simulink model "MCLV2_dsPIC33EP256MC506_externalOpAmp_DataLog"  (Simulink 9.2)
settings: Solver=FixedStepDiscrete  StartTime=0.0  StopTime=inf  FixedStep=Ts  RelTol=1e-3  EnableMultiTasking=on
PreLoadFcn:
  | InitTPV0;
undefined symbols (not defined in the file or in its folder): A4, A8, C5, C6, D5, F1, Lignes, NumBits1, NumBits2, P20, P24, P53, P54, P97, Pin, PWMmax, Slope1, Slope2, Timer, Tm, TPWM, TsQEI
undefined symbols (not defined in the file): Ts
libraries: simulink x16, MCHP_Blockset x14, simulink_need_slupdate x4, sl_helperblocks x1
(part 2 of 2)

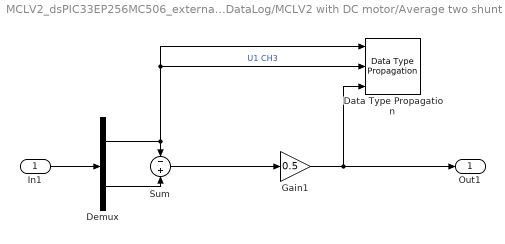
== system MCLV2_dsPIC33EP256MC506_externalOpAmp_DataLog/MCLV2 with DC motor/Average two shunt resistors ==
  In1 : Inport
  Data Type Propagation : simulink/Signal Attributes/Data Type Propagation  PropDataType=fixdt(1, 16)  IfRefDouble=double  IfRefSingle=single  IsSigned=IsSigned1 or IsSigned2  NumBitsBase=max([NumBits1 NumBits2])  NumBitsMult=1  NumBitsAdd=0  NumBitsAllowFinal=1:128  PropScaling=2^-10  ValuesUsedBestPrec=[5 -7]  SlopeBase=min([Slope1 Slope2])  SlopeMult=1  SlopeAdd=0  BiasBase=Bias1  BiasMult=1  BiasAdd=0
      settings: SourceProductName=Simulink  SourceProductBaseCode=SL
  Demux : Demux  Outputs=2
  Gain1 : Gain  Gain=0.5  ParamMin=[0.5]  ParamMax=[0.5]  OutDataTypeStr=Inherit: Inherit via back propagation  SaturateOnIntegerOverflow=on
  Sum : Sum  Inputs=-+  OutDataTypeStr=Inherit: Same as accumulator  SaturateOnIntegerOverflow=on
  Out1 : Outport
  wires:
  Demux/2 -> Sum/2
  Sum/1 -> Gain1/1
  Demux/1 -> Data Type Propagation/2, Data Type Propagation/1, Sum/1  "U1 CH3"
  In1/1 -> Demux/1
  Gain1/1 -> Data Type Propagation/3, Out1/1

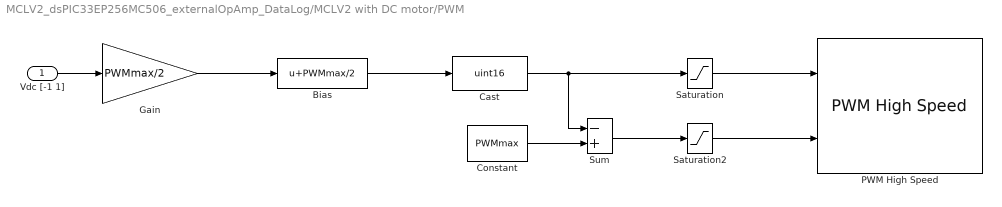
== system MCLV2_dsPIC33EP256MC506_externalOpAmp_DataLog/MCLV2 with DC motor/PWM ==
  Vdc [-1 1] : Inport
  Bias : Bias  Bias=PWMmax/2
  Cast : DataTypeConversion  OutDataTypeStr=uint16
  Constant : Constant  Value=PWMmax  OutDataTypeStr=uint16
  Gain : Gain  Gain=PWMmax/2  OutDataTypeStr=fixdt(1,32,1)
  PWM High Speed : MCHP_Blockset/PWM IO/PWM High Speed  pop1=[1]  chk1="[1  1  1  0  0]"  chkHL1="[1  1  0  1  1  1  1 ; 1  1  0  1  1  1  1]"  maxP1={ 'TPWM','0.001','0.001','0.001','0.001','0.001','0.001';'0.001','0.001','1e-06','0.001','0.001','0.001','0.001'}  InitP2={ 'TPWM','0.001','0.001','0.001','0.001','0.001','0.001';'0.001','0.001','0.001','0.001','0.001','0.001','0.001'}  chkP2="[0  1  0  1  1  1  1 ; 1  0  0  1  1  1  1]"  InitDC={ '50','50','50','50','50','50','50';'0.001','0.001','0.001','50','50','50','50'}  chkDC="[1  1  1  1  1  1  1 ; 0  0  0  1  1  1  1]"  InitPh={ '0','0','0','0.001','0.001','0.001','0.001';'0','0','0','0.001','0.001','0.001','0.001'}  chkPh="[0  0  0  1  1  1  1 ; 0  0  0  1  1  1  1]"  edSEvTrigx={ '0','-1','-1','-1','-1','-1','-1'}  chkSEvTrigx="[0  1  1  1  1  1  1]"  popFlt="[2  2  1  1  1  1  1]"  popFltPin="[20  20  20   4   4   4   4]"  popFltPinRp="[1  1  1  1  1  1  1]"  popFltActivH="[2  2  1  1  1  1  1]"  popFltForceH="[2  2  2  2  2  2  2]"  popFltForceL="[1  1  1  1  1  1  1]"  chkFltBlkOut="[0  0  0  0  0  0  0]"  popIndepFaultMode="[1  1  1  1  1  1  1]"  popCurEnabled="[1  1  1  1  1  1  1]"  popCurPin="[4  31   4   4   4   4   4]"  popCurActiveH="[1  1  1  1  1  1  1]"  popCurForceH="[2  1  2  1  1  1  1]"  popCurForceL="[2  1  2  1  1  1  1]"  ChkCurBlkOut="[1  0  0  0  0  0  0]"  ChkCurBlkOutTime="[1  0  1  0  0  0  0]"  popBLANKSEL="[1  1  1  1  1  1  1]"  popBPHHBPHL="[1  1  1  1  1  1  1]"  popBPLHBPLL="[1  1  1  1  1  1  1]"  popFLTLEBEN_CLLEBEN="[1  1  1  1  1  1  1]"  popPHR_PHF="[2  1  1  1  1  1  1]"  popPLR_PLF="[3  1  1  1  1  1  1]"  edLEB={ '100e-9','50e-9','150e-9','50e-9','50e-9','50e-9','50e-9'}  popDT="[1  1  1  3  3  3  3]"  edDTRx={ '0.02','1e-05','0.001','1e-05','1e-05','1e-05','1e-05'}  edAltDTRx={ 'Tm','Tm','Tm','1e-05','1e-05','1e-05','1e-05'}  S_INPUT="[5  5  5]"  S_INPUT_Size="[1  1  1]"  S_OUTPUT=[]  S_OUTPUT_Size=[]  S_DWORK_Type=[]  S_DWORK_Size=[]  ADC_VARTRIG={PWM Primary Special Event Trigger;6}  SampleTime=-1  ORDERING=None  MCHP_PORT={PWM1 Fault}{FLT32}4:0:B4;{PWM2 Fault}{FLT32}4:0:B4;{PWM1H}{PWM1H}4:4:B14;{PWM1L}{PWM1L}4:4:B15;{PWM2H}{PWM2H}4:4:B12;{PWM2L}{PWM2L}4:4:B13;  MCHP_MASTERLINK=MCLV2_dsPIC33EP256MC506_externalOpAmp_DataLog/Microchip Master  MCHP_VERSION=v3.39
      settings: SourceProductName=MPLAB® Device Blocks for Simulink®
  Saturation : Saturate  UpperLimit=PWMmax  LowerLimit=round( (Tm/TPWM) *PWMmax )
  Saturation2 : Saturate  UpperLimit=PWMmax  LowerLimit=round( (Tm/TPWM) *PWMmax )
  Sum : Sum  Inputs=-+  OutDataTypeStr=Inherit: Same as first input
  wires:
  Gain/1 -> Bias/1
  Cast/1 -> Sum/1, Saturation/1
  Saturation/1 -> PWM High Speed/1
  Sum/1 -> Saturation2/1
  Bias/1 -> Cast/1
  Saturation2/1 -> PWM High Speed/2
  Vdc [-1 1]/1 -> Gain/1
  Constant/1 -> Sum/2

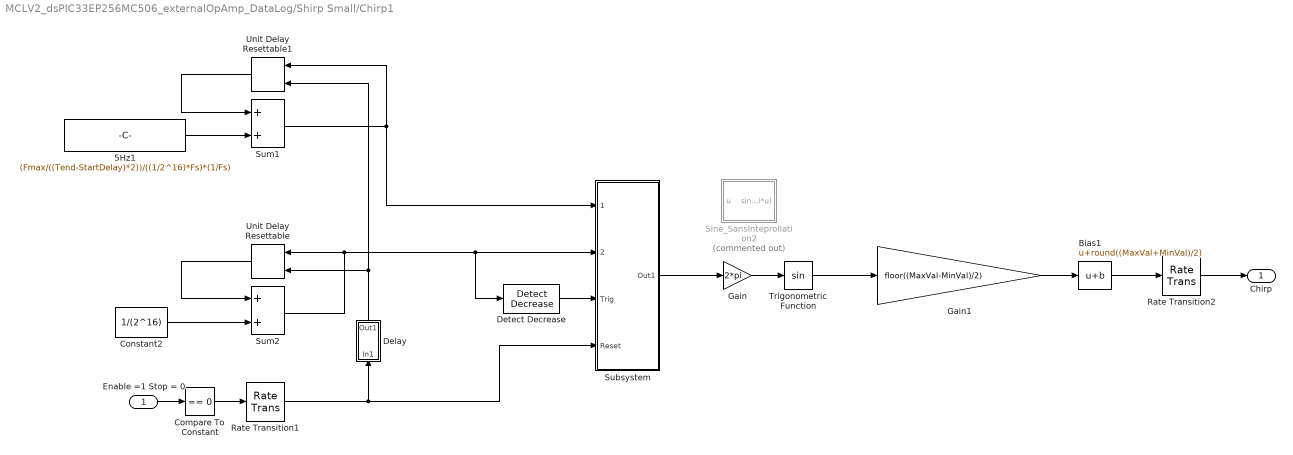
== system MCLV2_dsPIC33EP256MC506_externalOpAmp_DataLog/Shirp Small/Chirp1 ==
  Enable =1 Stop = 0 : Inport
  5Hz1 : Constant  Value=(Fmax/((Tend-StartDelay)*2))/((1/2^16)*Fs)*(1/Fs)  OutMin=(Fmax/((Tend-StartDelay)*2))/((1/2^16)*Fs)  OutMax=(Fmax/((Tend-StartDelay)*2))/((1/2^16)*Fs)  OutDataTypeStr=fixdt(0,32)  SampleTime=1/Fs
  Bias1 : Bias  Bias=round((MaxVal+MinVal)/2)
  Compare To Constant : simulink/Logic and Bit Operations/Compare To Constant  relop===  const=0  OutDataTypeStr=boolean
  Constant2 : Constant  Value=1/(2^16)  OutDataTypeStr=Inherit: Inherit via back propagation  SampleTime=1/Fs
  Delay : Subsystem
  Detect Decrease : simulink/Logic and Bit Operations/Detect Decrease  vinit=0.0  OutDataTypeStr=uint8
  Gain : Gain  Gain=2*pi  OutDataTypeStr=fixdt(0,16,13)
  Gain1 : Gain  Gain=floor((MaxVal-MinVal)/2)  OutMin=[MinVal]  OutMax=[MaxVal]  OutDataTypeStr=fixdt(MinVal<0,16)
  Rate Transition1 : RateTransition  Integrity=off  Deterministic=off
  Rate Transition2 : RateTransition  Integrity=off  Deterministic=off
  Sine_SansInteprollation2 : Subsystem  Commented=on  TreatAsAtomicUnit=on  mask(Sine and Cosine){Formula=sin(2*pi*u), NumDataPoints=(2^10)+1, OutputWordLength=16}
      mask prompts: Formula "Output formula"; NumDataPoints "Number of data points for lookup table:"; OutputWordLength "Output word length:"
      mask help:
      | Implement sine and cosine functions in fixed point using a lookup table approach that exploits quarter wave symmetry. The output fraction length equals the output word length minus 2.
      |
      | The most efficient implementation is obtained when the number of data points is (2^n)+1 where n is an integer.
      mask init:
      | if (~isnumeric(OutputWordLength)) || ( length(OutputWordLength) > 1 ) || ( OutputWordLength < 2 ) || ( floor(OutputWordLength) ~= OutputWordLength )
      |     error(DAStudio.message('Simulink:blocks:SineLookupWordLengthTooSmall'));
      | end
      | if (~isnumeric(NumDataPoints)) || ( length(NumDataPoints) > 1 ) || ( NumDataPoints < 2 ) || ( floor(NumDataPoints) ~= NumDataPoints )
      |     error(DAStudio.message('Simulink:blocks:SineLookupNumDataPtsTooSmall'));
      | end
      | if ( 2^(OutputWordLength-2) + 1 ) < NumDataPoints
      |     smallEnoughNumDataPoints = ( 2^(OutputWordLength-2) + 1 );
      |     bigEnoughOutputWordLength = ceil(log2(NumDataPoints-1))+2;
      |     error(DAStudio.message('Simulink:blocks:SineLookupEitherTooSmall',...
      |         NumDataPoints, ...
      |         smallEnoughNumDataPoints, ...
      |         OutputWordLength, ...
      |         bigEnoughOutputWordLength));
      | end
      | slsincos(Formula);
      mask TypeOptions Formula: sin(2*pi*u) | cos(2*pi*u) | exp(j*2*pi*u) | sin(2*pi*u) and cos(2*pi*u)
  Subsystem : Subsystem
  Sum1 : Sum  OutDataTypeStr=Inherit: Inherit via back propagation
  Sum2 : Sum  OutDataTypeStr=fixdt(0,16,16)
  Trigonometric Function : Trigonometry  ApproximationMethod=CORDIC
  Unit Delay Resettable : simulink_need_slupdate/Unit Delay Resettable  vinit=0.0  tsamp=inv(Fs)
      settings: SourceProductName=Simulink  SourceProductBaseCode=SL
  Unit Delay Resettable1 : simulink_need_slupdate/Unit Delay Resettable  vinit=0.0  tsamp=inv(Fs)
      settings: SourceProductName=Simulink  SourceProductBaseCode=SL
  Chirp : Outport
  wires:
  Gain/1 -> Trigonometric Function/1
  Trigonometric Function/1 -> Gain1/1
  Rate Transition1/1 -> Delay/1(In1), Subsystem/4(Reset)
  Rate Transition2/1 -> Chirp/1
  Enable =1 Stop = 0/1 -> Compare To Constant/1
  Compare To Constant/1 -> Rate Transition1/1
  Delay/1(Out1) -> Unit Delay Resettable1/2, Unit Delay Resettable/2
  Bias1/1 -> Rate Transition2/1
  Gain1/1 -> Bias1/1
  5Hz1/1 -> Sum1/2
  Unit Delay Resettable1/1 -> Sum1/1
  Sum1/1 -> Subsystem/1(Frequence), Unit Delay Resettable1/1
  Detect Decrease/1 -> Subsystem/3(Trig)
  Subsystem/1(Out1) -> Gain/1
  Constant2/1 -> Sum2/2
  Unit Delay Resettable/1 -> Sum2/1
  Sum2/1 -> Unit Delay Resettable/1, Subsystem/2(Compteur), Detect Decrease/1

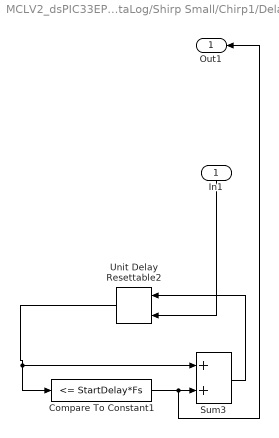
== system MCLV2_dsPIC33EP256MC506_externalOpAmp_DataLog/Shirp Small/Chirp1/Delay ==
  In1 : Inport
  Compare To Constant1 : simulink/Logic and Bit Operations/Compare To Constant  relop=<=  const=StartDelay*Fs  OutDataTypeStr=boolean
  Sum3 : Sum  AccumDataTypeStr=uint16  OutDataTypeStr=Inherit: Same as accumulator
  Unit Delay Resettable2 : simulink_need_slupdate/Unit Delay Resettable  vinit=1  tsamp=inv(Fs)
      settings: SourceProductName=Simulink  SourceProductBaseCode=SL
  Out1 : Outport
  wires:
  Unit Delay Resettable2/1 -> Sum3/1, Compare To Constant1/1
  Compare To Constant1/1 -> Sum3/2, Out1/1
  In1/1 -> Unit Delay Resettable2/2
  Sum3/1 -> Unit Delay Resettable2/1

== system MCLV2_dsPIC33EP256MC506_externalOpAmp_DataLog/Shirp Small/Chirp1/Sine_SansInteprollation2 ==
  u : Inport
  Sine : sl_helperblocks/Sine  NumDataPoints=NumDataPoints  OutputWordLength=OutputWordLength  InternalRulePriority=Precision
      settings: SourceProductName=Simulink  SourceProductBaseCode=SL
  sin(2*pi*u) : Outport
  wires:
  u/1 -> Sine/1
  Sine/1 -> sin(2*pi*u)/1

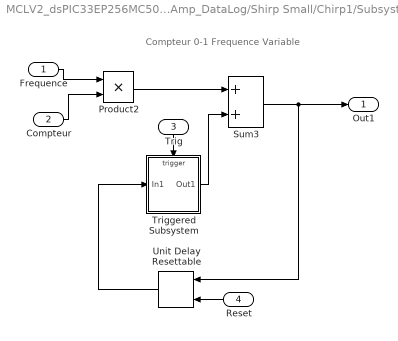
== system MCLV2_dsPIC33EP256MC506_externalOpAmp_DataLog/Shirp Small/Chirp1/Subsystem ==
  note: Compteur 0-1 Frequence Variable
  Frequence : Inport
  Compteur : Inport  Port=2
  Trig : Inport  Port=3
  Reset : Inport  Port=4
  Product2 : Product  OutDataTypeStr=fixdt(0,16,16)  RndMeth=Zero
  Sum3 : Sum  OutDataTypeStr=fixdt(0,16,16)
  Triggered Subsystem : Subsystem  TreatAsAtomicUnit=on
  Unit Delay Resettable : simulink_need_slupdate/Unit Delay Resettable  vinit=0.0  tsamp=inv(Fs)
      settings: SourceProductName=Simulink  SourceProductBaseCode=SL
  Out1 : Outport
  wires:
  Reset/1 -> Unit Delay Resettable/2
  Trig/1 -> Triggered Subsystem/Trigger
  Frequence/1 -> Product2/1
  Compteur/1 -> Product2/2
  Sum3/1 -> Unit Delay Resettable/1, Out1/1
  Unit Delay Resettable/1 -> Triggered Subsystem/1(In1)
  Triggered Subsystem/1(Out1) -> Sum3/2
  Product2/1 -> Sum3/1

== system MCLV2_dsPIC33EP256MC506_externalOpAmp_DataLog/Shirp Small/Chirp1/Subsystem/Triggered Subsystem ==
  In1 : Inport
  Trigger : TriggerPort  VariantControl=(inherit)
  Out1 : Outport
  wires:
  In1/1 -> Out1/1
